simulink model "gm_hdlcoderfftdit"  (R2016b)
settings: Solver=VariableStepDiscrete  StartTime=0.0  StopTime=15  RelTol=1e-3  EnableMultiTasking=on
InitFcn:
  | N=128;
  | Tcycle = 3*N/2-2 + log2(N)*(N/2+3);
  | 
  | if (N<=8)
  | Tcycle= Tcycle+1;
  | startLen = (ceil(Tcycle/N)+1)*N;
  | else
  | startLen = ceil(Tcycle/N)*N;
  | end
libraries: dspbuff3 x2, simulink x2, dspxfrm3 x1, simulink_need_slupdate x1, dspobslib x1, dspsrcs4 x1
settings Model: FPTRunName=Active  Creator=jma  LastModifiedBy=David Lavoie-Boutin
settings DataIOCC: LimitDataPoints=on  SaveFormat=Array  SaveOutput=off  SignalLogging=off  SaveTime=off
settings OptimizationCC: BlockReduction=off  ConditionallyExecuteInputs=off  ExpressionDepthLimit=2147483647  InitFltsAndDblsToZero=on  EfficientMapNaN2IntZero=off  LifeSpan=inf
settings DebuggingCC: UnderspecifiedInitializationDetection=Classic  MergeDetectMultiDrivingBlocksExec=none  SolverPrmCheckMsg=warning  InheritedTsInSrcMsg=none  IntegerOverflowMsg=none  ParameterOverflowMsg=warning  FcnCallInpInsideContextMsg=warning  StateNameClashWarn=warning  SFUnexpectedBacktrackingDiag=warning  SFNoUnconditionalDefaultTransitionDiag=warning  SFExecutionAtInitializationDiag=none  IntegerSaturationMsg=none
settings HardwareCC: ProdBitPerPointer=32  ProdBitPerSizeT=32  ProdBitPerPtrDiffT=32  ProdLargestAtomicFloat=None  ProdIntDivRoundTo=Undefined  ProdEndianess=Unspecified  ProdWordSize=32  ProdHWDeviceType=32-bit Generic
settings ModelReferenceCC: PropagateSignalLabelsOutOfModel=off
settings GRTTargetCC: TargetLangStandard=C89/C90 (ANSI)  GeneratePreprocessorConditionals=Disable all  CombineOutputUpdateFcns=off  GRTInterface=on
settings ConfigComp: CovMetricSettings=dw  CovHtmlReporting=on  CovSaveCumulativeToWorkspaceVar=on  CovSaveSingleToWorkspaceVar=on  CovExternalEMLEnable=off

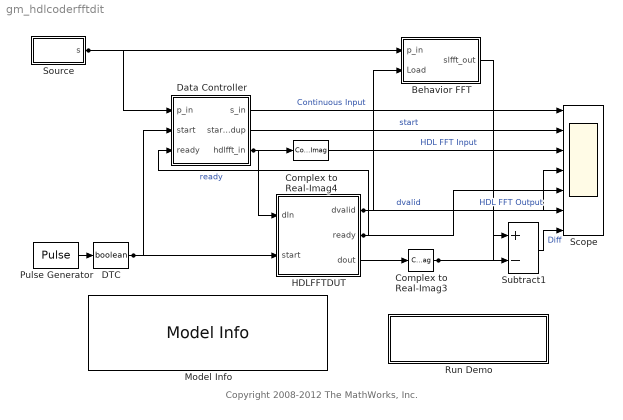
== system gm_hdlcoderfftdit ==
  note: Copyright 2008-2012 The MathWorks, Inc.
  Behavior FFT : Subsystem
  Complex to Real-Imag3 : ComplexToRealImag  Output=Real
  Complex to Real-Imag4 : ComplexToRealImag  Output=Real
  DTC : DataTypeConversion  OutDataTypeStr=boolean  RndMeth=Nearest  SaturateOnIntegerOverflow=on
  Data Controller : Subsystem
  HDLFFTDUT : Subsystem
  Model Info : simulink/Model-Wide Utilities/Model Info  Frame=on  DisplayStringWithTags=|  HorizontalTextAlignment=Center  LeftAlignmentValue=0.5  SourceBlockDiagram=gm_hdlcoderfftdit  TagMaxNumber=20
      | This demo shows how to use Simulink 
      | HDLCoder to check, generate, and verify 
      | HDL for a serial input serial output 
      | minimum resource architecture FFT model. 
      | Click the blue button to see the dialog.
  Pulse Generator : DiscretePulseGenerator  Period=startLen  PulseWidth=N/2  SampleTime=1/N
  Run Demo : Subsystem
      settings: OpenFcn=hdldialog(bdroot)
      mask Display: disp('Launch HDL Dialog')
  Scope : Scope  NumInputPorts=7
  Source : Subsystem
  Subtract1 : Sum  Inputs=+-  OutDataTypeStr=Inherit: Same as first input
  wires:
  Subtract1/1 -> Scope/7  "Diff"
  DTC/1 -> Data Controller/2(start), HDLFFTDUT/2(start)
  Data Controller/3(hdlfft_in) -> HDLFFTDUT/1(dIn), Complex to Real-Imag4/1
  Complex to Real-Imag3/1 -> Scope/6, Subtract1/2  "HDL FFT Output"
  HDLFFTDUT/3(dout) -> Complex to Real-Imag3/1
  HDLFFTDUT/2(ready) -> Scope/5, Data Controller/3(ready)  "ready"
  HDLFFTDUT/1(dvalid) -> Scope/4, Behavior FFT/2(Load)  "dvalid"
  Complex to Real-Imag4/1 -> Scope/3  "HDL FFT Input"
  Data Controller/2(start_dup) -> Scope/2  "start"
  Data Controller/1(s_in) -> Scope/1  "Continuous Input"
  Behavior FFT/1(slfft_out) -> Subtract1/1
  Pulse Generator/1 -> DTC/1
  Source/1(s) -> Data Controller/1(p_in), Behavior FFT/1(p_in)

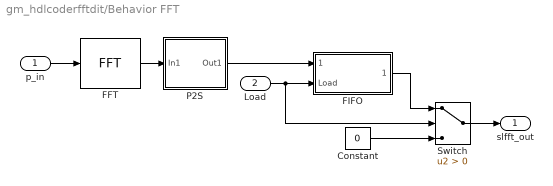
== system gm_hdlcoderfftdit/Behavior FFT ==
  p_in : Inport
  Load : Inport  Port=2
  Constant : Constant  Value=0  OutDataTypeStr=Inherit: Inherit via back propagation
  FFT : dspxfrm3/FFT  FFTImplementation=Auto  CompMethod=Table lookup  TableOpt=HYBRID  TableOptActive=Speed  BitRevOrder=off  Normalize=off  InheritFFTLength=on  FFTLength=64  WrapInput=on  roundingMode=Floor  overflowMode=on  firstCoeffDataTypeStr=Inherit: Same word length as input  firstCoeffLastDataTypeStr=Inherit: Same word length as input  outputMin=[]  outputMax=[]
  FIFO : Subsystem  TreatAsAtomicUnit=on
  P2S : Subsystem
  Switch : Switch  Criteria=u2 > Threshold
  slfft_out : Outport
  wires:
  Constant/1 -> Switch/3
  Switch/1 -> slfft_out/1
  Load/1 -> Switch/2, FIFO/2(Load)
  FIFO/1(SerialOut) -> Switch/1
  p_in/1 -> FFT/1
  P2S/1(Out1) -> FIFO/1(SerialIn)
  FFT/1 -> P2S/1(In1)

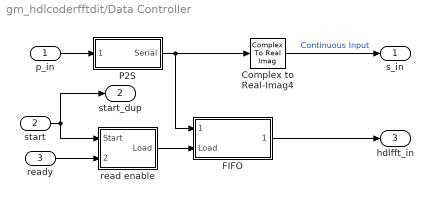
== system gm_hdlcoderfftdit/Data Controller ==
  p_in : Inport
  start : Inport  Port=2
  ready : Inport  Port=3
  Complex to Real-Imag4 : ComplexToRealImag  Output=Real
  FIFO : Subsystem  TreatAsAtomicUnit=on
  P2S : Subsystem
  read enable : Subsystem
  s_in : Outport
  start_dup : Outport  Port=2
  hdlfft_in : Outport  Port=3
  wires:
  Complex to Real-Imag4/1 -> s_in/1  "Continuous Input"
  ready/1 -> read enable/2(Ready)
  start/1 -> start_dup/1, read enable/1(Start)
  p_in/1 -> P2S/1(Parallel)
  P2S/1(Serial) -> FIFO/1(SerialIn), Complex to Real-Imag4/1
  read enable/1(Load) -> FIFO/2(Load)
  FIFO/1(SerialOut) -> hdlfft_in/1

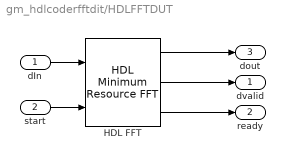
== system gm_hdlcoderfftdit/HDLFFTDUT ==
  dIn : Inport  OutDataTypeStr=int16  SampleTime=0.0078125
      settings: SignalType=complex
  start : Inport  Port=2  OutDataTypeStr=boolean  SampleTime=0.0078125
  HDL FFT : dspobslib/HDL Minimum Resource FFT  N=256  rnd=Floor  sat=Saturate  sinemode=Same word length as input  sineWL=10  prodmode=Same as input  prodWL=16  prodFL=13  accumode=Same as input  accuWL=18  accuFL=10  outputmode=Same as input  outputWL=16  outputFL=8
  dvalid : Outport
  ready : Outport  Port=2
  dout : Outport  Port=3
  wires:
  dIn/1 -> HDL FFT/1
  start/1 -> HDL FFT/2
  HDL FFT/1 -> dout/1
  HDL FFT/2 -> dvalid/1
  HDL FFT/3 -> ready/1

== system gm_hdlcoderfftdit/Run Demo ==

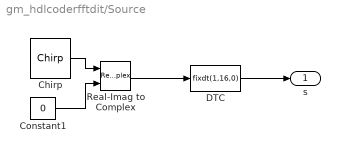
== system gm_hdlcoderfftdit/Source ==
  Chirp : dspsrcs4/Chirp  sweep=Linear  mode=Unidirectional  f0=2  f1=N/2  t1=1  Tsweep=10  phase=0  Ts=1/N  spf=N/8  datatype=Double  OutputFrames=on
  Constant1 : Constant  Value=0  OutDataTypeStr=Inherit: Inherit via back propagation
  DTC : DataTypeConversion  OutDataTypeStr=fixdt(1,16,0)  RndMeth=Nearest  SaturateOnIntegerOverflow=on
  Real-Imag to Complex : RealImagToComplex
  s : Outport
  wires:
  Real-Imag to Complex/1 -> DTC/1
  DTC/1 -> s/1
  Constant1/1 -> Real-Imag to Complex/2
  Chirp/1 -> Real-Imag to Complex/1

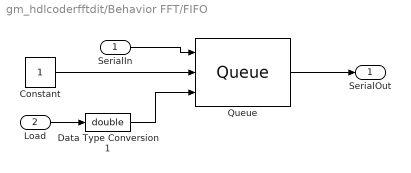
== system gm_hdlcoderfftdit/Behavior FFT/FIFO ==
  SerialIn : Inport
  Load : Inport  Port=2
  Constant : Constant
  Data Type Conversion1 : DataTypeConversion  OutDataTypeStr=double
  Queue : dspbuff3/Queue  depth=8*N  trigger=Non-zero sample  overflow=Dynamic reallocation  pes=Warning  eso=off  fso=off  nso=off  clr=off  clrOutport=off  adf=on
  SerialOut : Outport
  wires:
  SerialIn/1 -> Queue/1
  Constant/1 -> Queue/2
  Queue/1 -> SerialOut/1
  Load/1 -> Data Type Conversion1/1
  Data Type Conversion1/1 -> Queue/3

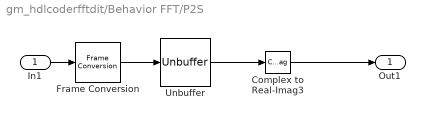
== system gm_hdlcoderfftdit/Behavior FFT/P2S ==
  In1 : Inport
  Complex to Real-Imag3 : ComplexToRealImag  Output=Real
  Frame Conversion : FrameConversion  InheritSamplingMode=off
  Unbuffer : Unbuffer  SampleBasedProcessing=Same as frame based
  Out1 : Outport
  wires:
  Complex to Real-Imag3/1 -> Out1/1
  In1/1 -> Frame Conversion/1
  Unbuffer/1 -> Complex to Real-Imag3/1
  Frame Conversion/1 -> Unbuffer/1

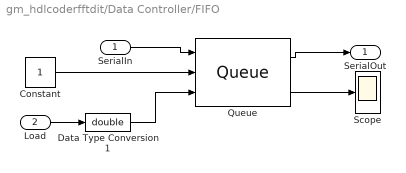
== system gm_hdlcoderfftdit/Data Controller/FIFO ==
  SerialIn : Inport
  Load : Inport  Port=2
  Constant : Constant
  Data Type Conversion1 : DataTypeConversion  OutDataTypeStr=double
  Queue : dspbuff3/Queue  depth=8*N  trigger=Non-zero sample  overflow=Dynamic reallocation  pes=Warning  eso=off  fso=on  nso=off  clr=off  clrOutport=off  adf=on
  Scope : Scope
  SerialOut : Outport
  wires:
  Queue/2 -> Scope/1
  Data Type Conversion1/1 -> Queue/3
  Load/1 -> Data Type Conversion1/1
  Queue/1 -> SerialOut/1
  Constant/1 -> Queue/2
  SerialIn/1 -> Queue/1

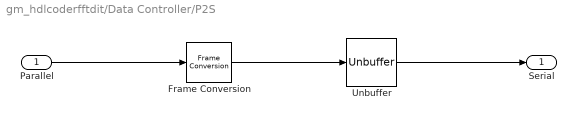
== system gm_hdlcoderfftdit/Data Controller/P2S ==
  Parallel : Inport
  Frame Conversion : FrameConversion  InheritSamplingMode=off
  Unbuffer : Unbuffer  SampleBasedProcessing=Same as frame based
  Serial : Outport
  wires:
  Parallel/1 -> Frame Conversion/1
  Frame Conversion/1 -> Unbuffer/1
  Unbuffer/1 -> Serial/1

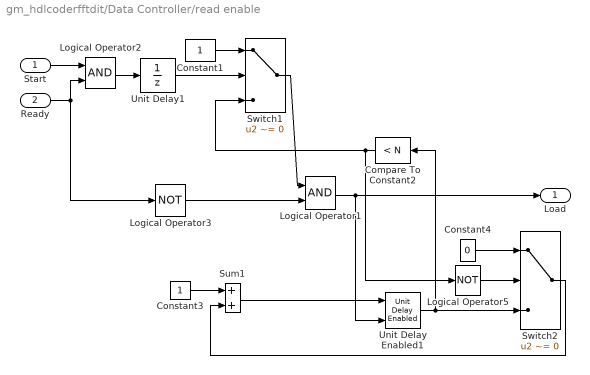
== system gm_hdlcoderfftdit/Data Controller/read enable ==
  Start : Inport
  Ready : Inport  Port=2
  Compare To Constant2 : simulink/Logic and Bit Operations/Compare To Constant  relop=<  const=N  OutDataTypeStr=boolean  ZeroCross=off
  Constant1 : Constant  OutDataTypeStr=uint32
  Constant3 : Constant  OutDataTypeStr=uint32
  Constant4 : Constant  Value=0  OutDataTypeStr=uint32
  Logical Operator1 : Logic  AllPortsSameDT=off  OutDataTypeStr=boolean
  Logical Operator2 : Logic  AllPortsSameDT=off  OutDataTypeStr=boolean
  Logical Operator3 : Logic  Operator=NOT  AllPortsSameDT=off  OutDataTypeStr=boolean
  Logical Operator5 : Logic  Operator=NOT  AllPortsSameDT=off  OutDataTypeStr=boolean
  Sum1 : Sum  OutDataTypeStr=uint32  RndMeth=Nearest  SaturateOnIntegerOverflow=on
  Switch1 : Switch  Criteria=u2 ~= 0
  Switch2 : Switch  Criteria=u2 ~= 0
  Unit Delay Enabled1 : simulink_need_slupdate/Unit Delay Enabled  vinit=0.0  tsamp=-1
  Unit Delay1 : UnitDelay  SampleTime=-1
  Load : Outport
  wires:
  Unit Delay1/1 -> Switch1/2
  Logical Operator5/1 -> Switch2/2
  Compare To Constant2/1 -> Logical Operator5/1, Switch1/3
  Ready/1 -> Logical Operator3/1, Logical Operator2/2
  Start/1 -> Logical Operator2/1
  Logical Operator3/1 -> Logical Operator1/2
  Switch1/1 -> Logical Operator1/1
  Constant1/1 -> Switch1/1
  Logical Operator2/1 -> Unit Delay1/1
  Logical Operator1/1 -> Unit Delay Enabled1/2, Load/1
  Switch2/1 -> Sum1/2
  Constant3/1 -> Sum1/1
  Sum1/1 -> Unit Delay Enabled1/1
  Unit Delay Enabled1/1 -> Compare To Constant2/1, Switch2/3
  Constant4/1 -> Switch2/1
